simulink model "reactor_feedback_observer"  (Simulink 10.2)
settings: Solver=ode15s  StartTime=0.0  StopTime=100  RelTol=1e-2  EnableMultiTasking=on
values from neighbouring files (symbols this model uses):
  A_linearized = [df1_dx1 df1_dx2 df1_dx3 df1_dx4;     df2_dx1 df2_dx2 df2_dx3 df2_dx4;     df3_dx1 df3_dx2 df3_dx3 df3_dx4;     df4_dx1 df4_dx2 df4_dx3 df4_dx4]    [assignment_q2.m]
  B_linearized = [df1_du1 df1_du2;     df2_du1 df2_du2;     df3_du1 df3_du2;     df4_du1 df4_du2]    [assignment_q2.m]
  C_est = [0 0 0 0; 0 0 0 0; 0 0 1 0; 0 0 0 1]    [assignment_q2.m]
  K = place(A_linearized, B_linearized, new_eig_values_K)    [assignment_q2.m]
  L = place(A_linearized', C_est', new_eig_values_L)'    [assignment_q2.m]
  u_s = [Fr_ss Qj_ss]    [assignment_q2.m]
undefined symbols (not defined in the file or in its folder): x_ss
settings Model: Creator=LemoineR  LastModifiedBy=mbatu
settings DataIOCC: LimitDataPoints=on
settings OptimizationCC: ExpressionDepthLimit=2147483647
settings DebuggingCC: SolverPrmCheckMsg=warning  AllowSymbolicDim=off  StateNameClashWarn=warning

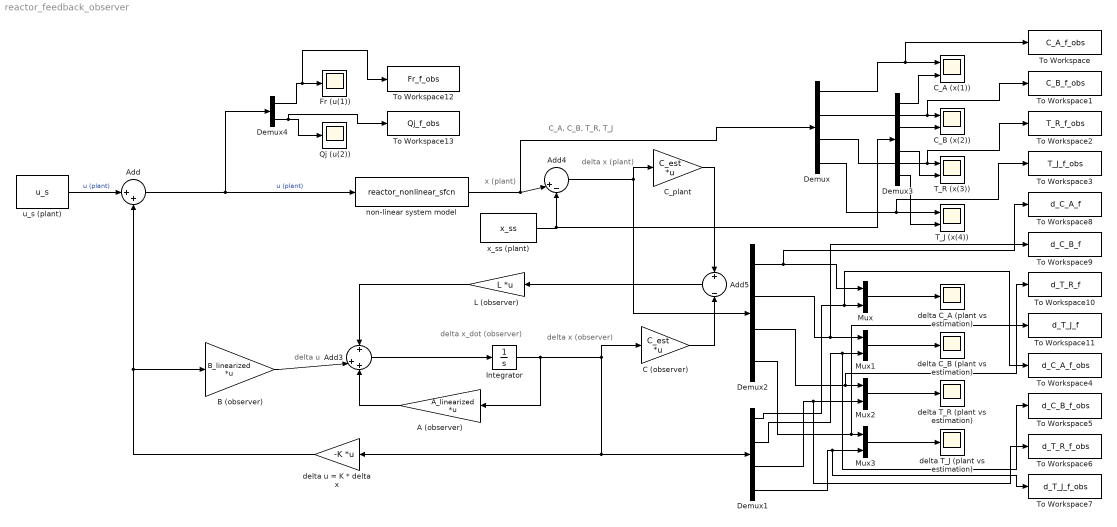
== system reactor_feedback_observer ==
  note: x (plant)
  note: delta x_dot
      | (observer)
  note: delta u
  note: delta x
      | (observer)
  note: C_A, C_B, T_R, T_J
  note: delta x
      | (plant)
  A (observer) : Gain  Gain=A_linearized  Multiplication=Matrix(K*u)
  Add : Sum  Inputs=|++
  Add3 : Sum  Inputs=+|++
  Add4 : Sum  Inputs=||+-
  Add5 : Sum  Inputs=+||-
  B (observer) : Gain  Gain=B_linearized  Multiplication=Matrix(K*u)
  C (observer) : Gain  Gain=C_est  Multiplication=Matrix(K*u)
  C_A (x(1)) : Scope  NumInputPorts=2
  C_B (x(2)) : Scope  NumInputPorts=2
  C_plant : Gain  Gain=C_est  Multiplication=Matrix(K*u)
  Demux{,1..3} (4 alike) : Demux
  Demux4 : Demux  Outputs=2
  Fr (u(1)) : Scope
  Integrator : Integrator
  L (observer) : Gain  Gain=L  Multiplication=Matrix(K*u)
  Mux{,1..3} (4 alike) : Mux  Inputs=2
  Qj (u(2)) : Scope
  T_J (x(4)) : Scope  NumInputPorts=2
  T_R (x(3)) : Scope  NumInputPorts=2
  To Workspace : ToWorkspace  VariableName=C_A_f_obs  SampleTime=-1
  To Workspace1 : ToWorkspace  VariableName=C_B_f_obs  SampleTime=-1
  To Workspace10 : ToWorkspace  VariableName=d_T_R_f  SampleTime=-1
  To Workspace11 : ToWorkspace  VariableName=d_T_J_f  SampleTime=-1
  To Workspace12 : ToWorkspace  VariableName=Fr_f_obs  SampleTime=-1
  To Workspace13 : ToWorkspace  VariableName=Qj_f_obs  SampleTime=-1
  To Workspace2 : ToWorkspace  VariableName=T_R_f_obs  SampleTime=-1
  To Workspace3 : ToWorkspace  VariableName=T_J_f_obs  SampleTime=-1
  To Workspace4 : ToWorkspace  VariableName=d_C_A_f_obs  SampleTime=-1
  To Workspace5 : ToWorkspace  VariableName=d_C_B_f_obs  SampleTime=-1
  To Workspace6 : ToWorkspace  VariableName=d_T_R_f_obs  SampleTime=-1
  To Workspace7 : ToWorkspace  VariableName=d_T_J_f_obs  SampleTime=-1
  To Workspace8 : ToWorkspace  VariableName=d_C_A_f  SampleTime=-1
  To Workspace9 : ToWorkspace  VariableName=d_C_B_f  SampleTime=-1
  delta C_A (plant vs estimation) : Scope
  delta C_B (plant vs estimation) : Scope
  delta T_J (plant vs estimation) : Scope
  delta T_R (plant vs estimation) : Scope
  delta u = K * delta x : Gain  Gain=-K  Multiplication=Matrix(K*u)
  non-linear system model : S-Function  FunctionName=reactor_nonlinear_sfcn  SFunctionDeploymentMode=off  EnableBusSupport=off
  u_s (plant) : Constant  Value=u_s
  x_ss (plant) : Constant  Value=x_ss
  wires:
  Demux/1 -> To Workspace/1, C_A (x(1))/1
  Demux/2 -> To Workspace1/1, C_B (x(2))/1
  Add/1 -> Demux4/1, non-linear system model/1  "u (plant)"
  Add3/1 -> Integrator/1
  Integrator/1 -> C (observer)/1, delta u = K * delta x/1, Demux1/1, A (observer)/1
  non-linear system model/1 -> Add4/1, Demux/1
  x_ss (plant)/1 -> Add4/2, Demux3/1
  Add4/1 -> Demux2/1, C_plant/1
  C (observer)/1 -> Add5/2
  Add5/1 -> L (observer)/1
  B (observer)/1 -> Add3/2
  A (observer)/1 -> Add3/3
  L (observer)/1 -> Add3/1
  Demux1/2 -> Mux1/2, To Workspace5/1
  Mux/1 -> delta C_A (plant vs estimation)/1
  Mux1/1 -> delta C_B (plant vs estimation)/1
  Demux2/1 -> Mux/1, To Workspace8/1
  Demux2/2 -> Mux1/1, To Workspace9/1
  Demux4/2 -> To Workspace13/1, Qj (u(2))/1
  Demux4/1 -> To Workspace12/1, Fr (u(1))/1
  Demux/3 -> To Workspace2/1, T_R (x(3))/1
  Demux/4 -> To Workspace3/1, T_J (x(4))/1
  Mux2/1 -> delta T_R (plant vs estimation)/1
  Mux3/1 -> delta T_J (plant vs estimation)/1
  Demux2/3 -> To Workspace10/1, Mux2/1
  Demux1/3 -> Mux2/2, To Workspace6/1
  Demux2/4 -> To Workspace11/1, Mux3/1
  Demux1/4 -> To Workspace7/1, Mux3/2
  C_plant/1 -> Add5/1
  delta u = K * delta x/1 -> B (observer)/1, Add/2
  u_s (plant)/1 -> Add/1  "u (plant)"
  Demux3/2 -> C_B (x(2))/2
  Demux3/1 -> C_A (x(1))/2
  Demux3/3 -> T_R (x(3))/2
  Demux3/4 -> T_J (x(4))/2
  Demux1/1 -> To Workspace4/1, Mux/2
